simulink model "transfer_function_structured"  (R2023a)
settings: Solver=VariableStepAuto  StartTime=0.0  StopTime=10.0  RelTol=1e-3
undefined symbols (not defined in the file or in its folder): G_D_sim_denominator_1, G_D_sim_denominator_2, G_D_sim_numerator_1, G_D_sim_numerator_2, G_S_sim_denominator_11, G_S_sim_denominator_12, G_S_sim_denominator_21, G_S_sim_denominator_22, G_S_sim_numerator_11, G_S_sim_numerator_12, G_S_sim_numerator_21, G_S_sim_numerator_22
settings Model: Creator=pascalbock  LastModifiedBy=pascalbock

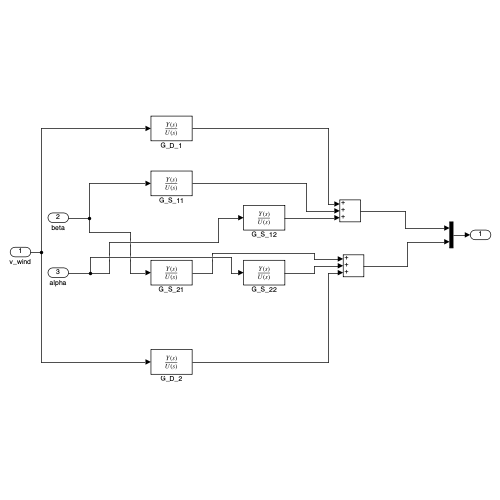
[thumbnail: Simulink's stored preview of the top-level diagram]
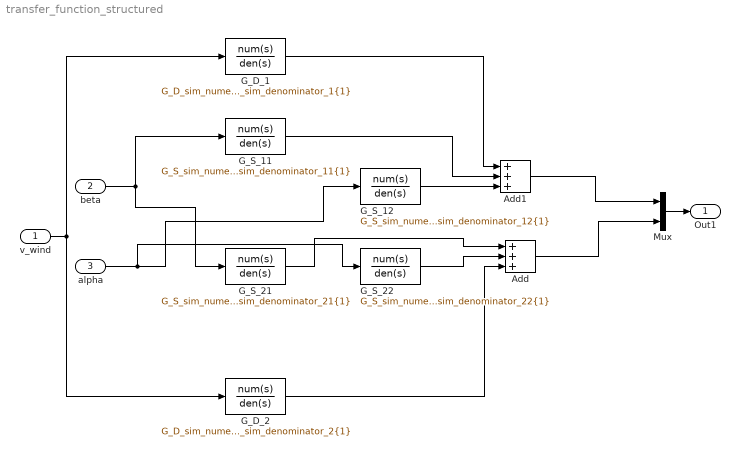
== system transfer_function_structured ==
  v_wind : Inport
  beta : Inport  Port=2
  alpha : Inport  Port=3
  Add : Sum  Inputs=+++
  Add1 : Sum  Inputs=+++
  G_D_1 : TransferFcn  Numerator=G_D_sim_numerator_1{1}  Denominator=G_D_sim_denominator_1{1}
  G_D_2 : TransferFcn  Numerator=G_D_sim_numerator_2{1}  Denominator=G_D_sim_denominator_2{1}
  G_S_11 : TransferFcn  Numerator=G_S_sim_numerator_11{1}  Denominator=G_S_sim_denominator_11{1}
  G_S_12 : TransferFcn  Numerator=G_S_sim_numerator_12{1}  Denominator=G_S_sim_denominator_12{1}
  G_S_21 : TransferFcn  Numerator=G_S_sim_numerator_21{1}  Denominator=G_S_sim_denominator_21{1}
  G_S_22 : TransferFcn  Numerator=G_S_sim_numerator_22{1}  Denominator=G_S_sim_denominator_22{1}
  Mux : Mux  Inputs=2
  Out1 : Outport
  wires:
  alpha/1 -> G_S_22/1, G_S_12/1
  G_S_12/1 -> Add1/3
  v_wind/1 -> G_D_2/1, G_D_1/1
  G_D_1/1 -> Add1/1
  G_S_11/1 -> Add1/2
  Add/1 -> Mux/2
  G_S_21/1 -> Add/1
  G_S_22/1 -> Add/2
  G_D_2/1 -> Add/3
  Add1/1 -> Mux/1
  Mux/1 -> Out1/1
  beta/1 -> G_S_11/1, G_S_21/1
